simulink model "obiekt"  (Simulink 7.4)
settings: Solver=ode3  StartTime=0.0  StopTime=10.0  FixedStep=1e-02  RelTol=1e-3
values from neighbouring files (symbols this model uses):
  iS = abs(ceil((randn * 10)+10))    [TestujObiekt.m]
  L = [3]    [Symuluj.m]
  M = [2, 1, 1]    [Symuluj.m]
  SPS = 10    [Symuluj.m]
  T = [0: 1/SPS : N/SPS - 1/SPS]    [GeneratorWeWy.m]    (also in Skok.m; Symuluj.m = 0.3)
settings Model: Creator=Konrad  LastModifiedBy=Konrad

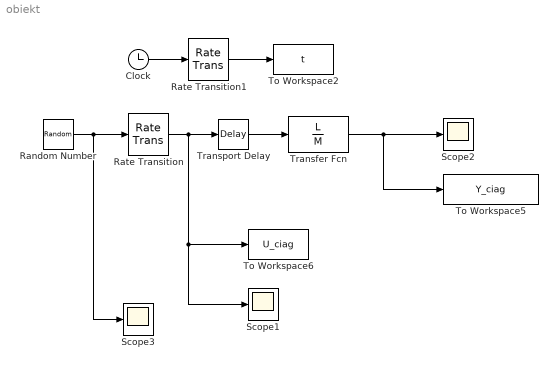
== system obiekt ==
  Clock : Clock
      settings: Decimation=10
  Random Number : RandomNumber  Variance=200000  Seed=iS  SampleTime=2
  Rate Transition : RateTransition
  Rate Transition1 : RateTransition  OutPortSampleTime=1/SPS
  Scope1 : Scope
  Scope2 : Scope
  Scope3 : Scope
      settings: SaveName=ScopeData2
  To Workspace2 : ToWorkspace  VariableName=t  SampleTime=1/SPS  SaveFormat=Array
  To Workspace5 : ToWorkspace  VariableName=Y_ciag  SampleTime=-1  SaveFormat=Array
  To Workspace6 : ToWorkspace  VariableName=U_ciag  SampleTime=-1  SaveFormat=Array
  Transfer Fcn : TransferFcn  Numerator=L  Denominator=M
  Transport Delay : TransportDelay  DelayTime=T
  wires:
  Clock/1 -> Rate Transition1/1
  Transfer Fcn/1 -> Scope2/1, To Workspace5/1
  Transport Delay/1 -> Transfer Fcn/1
  Rate Transition/1 -> To Workspace6/1, Scope1/1, Transport Delay/1
  Rate Transition1/1 -> To Workspace2/1
  Random Number/1 -> Rate Transition/1, Scope3/1
